simulink model "ES101A_DiagcMgr"  (R2013b)
settings: Solver=ode45  StartTime=0.0  StopTime=0.44  RelTol=1e-3
values from neighbouring files (symbols this model uses):
  BrdgVltg = DataDict.IpSignal    [ES101A_DiagcMgr_DataDict.m]
  DEM_CLEAR_PENDING = DataDict.Constant    [ES101A_DiagcMgr_DataDict.m]
  DEM_DTC_GROUP_ALL_DTCS = DataDict.Constant    [ES101A_DiagcMgr_DataDict.m]
  DFTAGICNTR_CNT_U08 = DataDict.Constant    [ES101A_DiagcMgr_DataDict.m]
  DIAGCMGR_NTCINFOSTSTESTFAILD_CNT_U08 = DataDict.Constant    [ES101A_DiagcMgrProxyX_DataDict.m]    (also in ES101A_DiagcMgr_DataDict.m)
  DIAGCMGR_NTCINFOSTSTESTFAILDTHISIGNCYC_CNT_U08 = DataDict.Constant    [ES101A_DiagcMgr_DataDict.m]
  DIAGCMGR_NTCINFOSTSTESTNOTCMPLTHISIGNCYC_CNT_U08 = DataDict.Constant    [ES101A_DiagcMgrProxyX_DataDict.m]    (also in ES101A_DiagcMgr_DataDict.m)
  DiagcMgrFltResp = DataDict.Calibration    [ES101A_DiagcMgrProxyX_DataDict.m]    (also in ES101A_DiagcMgr_DataDict.m)
  DiagcMgrNtcFltAry = DataDict.NVM    [ES101A_DiagcMgr_DataDict.m]
  DIAGCSTSCTRLDSHTDWNFLTPRSNT_CNT_U16 = DataDict.Constant    [ES101A_DiagcMgr_DataDict.m]
  DIAGCSTSDFTHWAG_CNT_U16 = DataDict.Constant    [ES101A_DiagcMgr_DataDict.m]
  DIAGCSTSDFTHWAGSERLCOMEXPRTVAL_CNT_U16 = DataDict.Constant    [ES101A_DiagcMgr_DataDict.m]
  DIAGCSTSDFTVEHSPD_CNT_U16 = DataDict.Constant    [ES101A_DiagcMgr_DataDict.m]
  DIAGCSTSININVAL_CNT_U16 = DataDict.Constant    [ES101A_DiagcMgrProxyX_DataDict.m]    (also in ES101A_DiagcMgr_DataDict.m)
  DIAGCSTSIVTR1INACTV_CNT_U16 = DataDict.Constant    [ES101A_DiagcMgr_DataDict.m]
  DIAGCSTSIVTR2INACTV_CNT_U16 = DataDict.Constant    [ES101A_DiagcMgr_DataDict.m]
  DIAGCSTSLIMDTPRFMNC_CNT_U16 = DataDict.Constant    [ES101A_DiagcMgr_DataDict.m]
  DIAGCSTSRAMPTOZEROFLTPRSNT_CNT_U16 = DataDict.Constant    [ES101A_DiagcMgr_DataDict.m]
  DIAGCSTSWHLIMBREJCTNDI_CNT_U16 = DataDict.Constant    [ES101A_DiagcMgr_DataDict.m]
  DTCIDXSTSFAIL_CNT_U08 = DataDict.Constant    [ES101A_DiagcMgr_DataDict.m]
  DTCIDXSTSNONTC_CNT_U08 = DataDict.Constant    [ES101A_DiagcMgr_DataDict.m]
  DTCIDXSTSNORES_CNT_U08 = DataDict.Constant    [ES101A_DiagcMgr_DataDict.m]
  DTCIDXSTSPASS_CNT_U08 = DataDict.Constant    [ES101A_DiagcMgr_DataDict.m]
  DTCIDXSTSUPDCFMD_CNT_U08 = DataDict.Constant    [ES101A_DiagcMgr_DataDict.m]
  ELECGLBPRM_IVTRCNT_CNT_U08 = DataDict.ConfigParam    [ES101A_DiagcMgrProxyX_DataDict.m]    (also in ES101A_DiagcMgr_DataDict.m)
  FLTINJ_DIAGCMGR_DIAGCSTSIVTR1INACTV = DataDict.Constant    [ES101A_DiagcMgr_DataDict.m]
  FLTINJ_DIAGCMGR_DIAGCSTSIVTR2INACTV = DataDict.Constant    [ES101A_DiagcMgr_DataDict.m]
  HwTq = DataDict.IpSignal    [ES101A_DiagcMgr_DataDict.m]
  IgnCntr = DataDict.IpSignal    [ES101A_DiagcMgr_DataDict.m]
  MAXDEBCNTRVAL_CNT_S16 = DataDict.Constant    [ES101A_DiagcMgr_DataDict.m]
  MAXRAMPRATE_ULSPERSEC_F32 = DataDict.Constant    [ES101A_DiagcMgrProxyX_DataDict.m]    (also in ES101A_DiagcMgr_DataDict.m)
  MINDEBCNTRVAL_CNT_S16 = DataDict.Constant    [ES101A_DiagcMgr_DataDict.m]
  MINRAMPRATE_ULSPERSEC_F32 = DataDict.Constant    [ES101A_DiagcMgrProxyX_DataDict.m]    (also in ES101A_DiagcMgr_DataDict.m)
  SCAMOTTQCMDTOONE_ULS_F32 = DataDict.Constant    [ES101A_DiagcMgrProxyX_DataDict.m]    (also in ES101A_DiagcMgr_DataDict.m)
  SCAMOTTQCMDTOZERO_ULS_F32 = DataDict.Constant    [ES101A_DiagcMgrProxyX_DataDict.m]    (also in ES101A_DiagcMgr_DataDict.m)
  SysSt = DataDict.IpSignal    [ES101A_DiagcMgr_DataDict.m]
  VehSpd = DataDict.IpSignal    [ES101A_DiagcMgr_DataDict.m]
undefined symbols (not defined in the file or in its folder): ActvMotTqCmdSca, ActvRampRate, AgiCntr, Dem_DTCFormatType, Dem_DTCOriginType, Dem_EventStatusType, DiagcData, DiagcMgrNtcMap, DiagcSts, DtcEnaMask, EcuT, HistNtcFltAry, MicroDiagcData, MotTq, NtcNr, NtcNrWithResd1, NtcStInfo, ProxySetNtcData, Sts, SysSt1, TOTNROFDTC_CNT_U08
libraries: simulink x149, FloatToFixd x5, NxtrNvM x3
(part 8 of 13)

== system ES101A_DiagcMgr/DiagcMgr/SetNtcStsCore/NtcNr is Valid/Diagnostics Not Inhibited/NtcEnabled/NTCSTS_PREFAILD/Update NtcInfoSts, DebCntr and Process RampRate ==
  NtcInfo_ArgIn : Inport
  DebStep_ArgIn : Inport  Port=2
  NtcStInfo_ArgIn : Inport  Port=3
  NtcNr_ArgIn : Inport  Port=4
  DiagcData_ArgIn : Inport  Port=5
  ProxySetNtcData_ArgIn : Inport  Port=6
  NtcInfoDebCntr_ArgIn : Inport  Port=7
  SnapshotDataBus : Inport  Port=8
  Constant : Constant  Value=MAXDEBCNTRVAL_CNT_S16
  CopyRight2 : Subsystem  Description=|  mask(Copyright Information){none=on}
      | Copyright info block.                                               
      |                                                                     
      | Place copyright information at the top of every subsystem in design.
      mask prompts: none "No parameters"
      mask help: Place copyright information at the top of every subsystem in design.
      mask Display:
      | NxtrConf = 'Nexteer Confidential';
      | 
      | sys = bdroot; %handle for the current model ("system")
      | first = get_param(sys,'Created');
      | first = first(end-3:end);  %year is last four digits
      | 
      | last = get_param(sys,'LastModifiedDate');
      | if isempty(last)
      |     last = datestr(now,'yyyy');
      | else
      |     last = last(end-3:end);
      | end
      | 
      | if strcmp(first,last)
      |     fprintf('%s -- Copyright %s Nexteer',NxtrConf,first)
      | else
      |     fprintf('%s -- %s%s- %s Nexteer',NxtrConf,char(169),first,last)
      | end
  Deb Counter < MAXDEBCNTRVAL_CNT_S16 : Subsystem  RequirementInfo="{'linktype_rmi_doors' '0000c474 (/ESG Group/FDD Module Requirements/EA4 Specific/ES101A_DiagcMgr)' '#ES101A_275' 'true' 'REQ:  ES101A_275' '' ; 'linktype_rmi_doors' '0000c474 (/ESG Group/FDD Module Requirements/EA4 Specific/ES101A_DiagcMgr)' '#ES101A_277' 'true' 'REQ:  ES101A_277' '' } %GIDa_78053276_d02e_468e_a567_0a861c97d8c0"  TreatAsAtomicUnit=on
  DebCntr = MAXDEBCNTRVAL_CNT_S16 : Subsystem  TreatAsAtomicUnit=on
  If1 : If  NumInputs=3  IfExpression="(u1 >=  u2) | (u3 >= 32767)"
  Merge1 : Merge
  Sub1 : Sum  Inputs=-+  SaturateOnIntegerOverflow=on
  NtcInfo_ArgOut : Outport
  DiagcData_ArgOut : Outport  Port=2
  NtcInfoDebCntr_ArgOut : Outport  Port=3
  ProxySetNtcData_ArgOut : Outport  Port=4
  wires:
  If1/1 -> DebCntr = MAXDEBCNTRVAL_CNT_S16/Action
  If1/2 -> Deb Counter < MAXDEBCNTRVAL_CNT_S16/Action
  NtcInfo_ArgIn/1 -> Deb Counter < MAXDEBCNTRVAL_CNT_S16/1(NtcInfoDebCntr_ArgIn), DebCntr = MAXDEBCNTRVAL_CNT_S16/5(NtcInfo_ArgIn)
  Constant/1 -> Sub1/2
  Sub1/1 -> If1/2
  Deb Counter < MAXDEBCNTRVAL_CNT_S16/1(NtcInfoDebCntr_ArgOut) -> Merge1/2
  DebCntr = MAXDEBCNTRVAL_CNT_S16/4(NtcInfoDebCntr_ArgOut) -> Merge1/1
  Merge1/1 -> NtcInfoDebCntr_ArgOut/1
  NtcStInfo_ArgIn/1 -> DebCntr = MAXDEBCNTRVAL_CNT_S16/4(NtcStInfo_ArgIn)
  ProxySetNtcData_ArgIn/1 -> DebCntr = MAXDEBCNTRVAL_CNT_S16/3(ProxySetNtcData_ArgIn)
  DiagcData_ArgIn/1 -> DebCntr = MAXDEBCNTRVAL_CNT_S16/2(DiagcData_ArgIn)
  NtcNr_ArgIn/1 -> DebCntr = MAXDEBCNTRVAL_CNT_S16/1(NtcNr_ArgIn)
  DebCntr = MAXDEBCNTRVAL_CNT_S16/1(DiagcData_ArgOut) -> DiagcData_ArgOut/1
  DebCntr = MAXDEBCNTRVAL_CNT_S16/2(ProxySetNtcData_ArgOut) -> ProxySetNtcData_ArgOut/1
  NtcInfoDebCntr_ArgIn/1 -> If1/1
  DebCntr = MAXDEBCNTRVAL_CNT_S16/3(NtcInfo_ArgOut) -> NtcInfo_ArgOut/1
  SnapshotDataBus/1 -> DebCntr = MAXDEBCNTRVAL_CNT_S16/6(SnapshotDataBus)
  DebStep_ArgIn/1 -> Sub1/1, If1/3, Deb Counter < MAXDEBCNTRVAL_CNT_S16/2(DebStep_ArgIn)

== system ES101A_DiagcMgr/DiagcMgr/SetNtcStsCore/NtcNr is Valid/Diagnostics Not Inhibited/NtcEnabled/NTCSTS_PREPASSD/CopyRight2 ==

== system ES101A_DiagcMgr/DiagcMgr/SetNtcStsCore/NtcNr is Valid/Diagnostics Not Inhibited/NtcEnabled/NTCSTS_PREPASSD/Update NtcInfoSts ==
  NtcNr_ArgIn : Inport
  DebStep_ArgIn : Inport  Port=2
  NtcInfo_ArgIn : Inport  Port=3
  NtcInfoDebCntr_ArgIn : Inport  Port=4
  " DIAGCMGR_NTCINFOSTSTESTFAILDTHISIGNCYC_CNT_U08" : simulink/Logic and Bit Operations/Bitwise Operator  logicop=AND  UseBitMask=on  BitMask=DIAGCMGR_NTCINFOSTSTESTFAILDTHISIGNCYC_CNT_U08  BitMaskRealWorld=Stored Integer
  Bus Selector : BusSelector  OutputSignals=Sts
  CopyRight2 : Subsystem  Description=|  mask(Copyright Information){none=on}
      | Copyright info block.                                               
      |                                                                     
      | Place copyright information at the top of every subsystem in design.
      mask prompts: none "No parameters"
      mask help: Place copyright information at the top of every subsystem in design.
      mask Display:
      | NxtrConf = 'Nexteer Confidential';
      | 
      | sys = bdroot; %handle for the current model ("system")
      | first = get_param(sys,'Created');
      | first = first(end-3:end);  %year is last four digits
      | 
      | last = get_param(sys,'LastModifiedDate');
      | if isempty(last)
      |     last = datestr(now,'yyyy');
      | else
      |     last = last(end-3:end);
      | end
      | 
      | if strcmp(first,last)
      |     fprintf('%s -- Copyright %s Nexteer',NxtrConf,first)
      | else
      |     fprintf('%s -- %s%s- %s Nexteer',NxtrConf,char(169),first,last)
      | end
  Data Type Conversion : DataTypeConversion  OutDataTypeStr=boolean
  Data Type Conversion1 : DataTypeConversion  OutDataTypeStr=boolean
  Data Type Conversion2 : DataTypeConversion  OutDataTypeStr=uint16
  Do Nothing : Subsystem
  FLTRESPRCVRLFLT_CNT_U32 : simulink/Logic and Bit Operations/Bitwise Operator  logicop=AND  UseBitMask=on  BitMask=FLTRESPRCVRLFLT_CNT_U32  BitMaskRealWorld=Stored Integer
  Fault Response Table : Constant  Value=DiagcMgrFltResp
  If : If  NumInputs=2  IfExpression=(u1 == 1)|(u2 == 0)
  Selector1 : Selector  IndexMode=Zero-based  InputPortWidth=512  IndexOptions=Index vector (port)  Indices=[1 3]  OutputSizes=1
  Update NTC Info's Status Byte & Update the NTC Fault Array : Subsystem  RequirementInfo="{'linktype_rmi_doors' '0000c474 (/ESG Group/FDD Module Requirements/EA4 Specific/ES101A_DiagcMgr)' '#ES101A_193' 'true' 'REQ:  ES101A_193' '' ; 'linktype_rmi_doors' '0000c474 (/ESG Group/FDD Module Requirements/EA4 Specific/ES101A_DiagcMgr)' '#ES101A_253' 'true' 'REQ:  ES101A_253' '' ; 'linktype_rmi_doors' '0000c474 (/ESG Group/FDD Module Requirements/EA4 Specific/ES101A_DiagcMgr)' '#ES101A_194' 'true' 'REQ:  ES101A_194' '' ; 'linktype_rmi_doors' '0000c474 (/ESG Group/FDD Module Requirements/EA4 Specific/ES101A_DiagcMgr)' '#ES101A_195' 'true' 'REQ:  ES101A_195' '' } %GIDa_8b4eb5db_0f86_4d26_94c4_2021364c827d"
  NtcInfo_ArgOut : Outport
  NtcInfoDebCntr_ArgOut : Outport  Port=2
  wires:
  Data Type Conversion2/1 -> Selector1/2
  Update NTC Info's Status Byte & Update the NTC Fault Array/1("NtcInfo_ArgOut ") -> NtcInfo_ArgOut/1
  Data Type Conversion1/1 -> If/2
  " DIAGCMGR_NTCINFOSTSTESTFAILDTHISIGNCYC_CNT_U08"/1 -> Data Type Conversion1/1
  Bus Selector/1 -> " DIAGCMGR_NTCINFOSTSTESTFAILDTHISIGNCYC_CNT_U08"/1  "<Sts>"
  NtcInfo_ArgIn/1 -> Update NTC Info's Status Byte & Update the NTC Fault Array/1(NtcInfo_ArgIn), Bus Selector/1
  DebStep_ArgIn/1 -> Update NTC Info's Status Byte & Update the NTC Fault Array/2(DebStep_ArgIn)
  If/2 -> Do Nothing/Action
  If/1 -> Update NTC Info's Status Byte & Update the NTC Fault Array/Action
  Data Type Conversion/1 -> If/1
  FLTRESPRCVRLFLT_CNT_U32/1 -> Data Type Conversion/1
  Fault Response Table/1 -> Selector1/1
  Selector1/1 -> FLTRESPRCVRLFLT_CNT_U32/1
  NtcNr_ArgIn/1 -> Data Type Conversion2/1
  NtcInfoDebCntr_ArgIn/1 -> Update NTC Info's Status Byte & Update the NTC Fault Array/3(NtcInfoDebCntr_ArgIn)
  Update NTC Info's Status Byte & Update the NTC Fault Array/2(NtcInfoDebCntr_ArgOut) -> NtcInfoDebCntr_ArgOut/1

== system ES101A_DiagcMgr/DiagcMgr/DiagcMgrIninCore/Update NtcInfoAry From NvM/Update NtcInfoAry/Update NtcInfoAry Aging Counter And Confirmed Bit/If Action/Subsystem/0 < AgingCntr < 64 ==
  note: SW Implementation:
      |
      | 	Design is generalized with the use of "DiagcMgrNtcInfoX" as the NtcInfoAry. When the NTC from the NvM is read
      | 	and it is looked up against the NtcMap to find its ApplIdx and NtcInfoIdx. ApplIdx indicates which NtcInfo the NTC
      | 	belongs to. NtcInfoIdx is used to find the NtcInfo data corresponding to that NTC in the NtcInfoIdx.
      |
      | 	This design does not show which NtcInfoAry does an NTC belong to, instead shows a generalized NtcInfoX.
      | 	The software implementaion shall use the ApplIdx to index into the correct NtcInfoAry and then used the NtcInfoIdx
      | 	to index into the correct data for any NTC.
  NtcNr : Inport
  AgiCntr : Inport  Port=2
  "Sts " : Inport  Port=3
  NtcInfoAry_ArgIn : Inport  Port=4
  Action Port : ActionPort
  Assignment : Assignment  IndexMode=Zero-based  IndexOptions=Index vector (port)  Indices=1  OutputSizes=1
  Bus Assignment1 : BusAssignment  AssignedSignals=Sts,AgiCntr
  Bus Selector2 : BusSelector  OutputSignals=ApplIdx,NtcInfoIdx
  CopyRight2 : Subsystem  Description=|  mask(Copyright Information){none=on}
      | Copyright info block.                                               
      |                                                                     
      | Place copyright information at the top of every subsystem in design.
      mask prompts: none "No parameters"
      mask help: Place copyright information at the top of every subsystem in design.
      mask Display:
      | NxtrConf = 'Nexteer Confidential';
      | 
      | sys = bdroot; %handle for the current model ("system")
      | first = get_param(sys,'Created');
      | first = first(end-3:end);  %year is last four digits
      | 
      | last = get_param(sys,'LastModifiedDate');
      | if isempty(last)
      |     last = datestr(now,'yyyy');
      | else
      |     last = last(end-3:end);
      | end
      | 
      | if strcmp(first,last)
      |     fprintf('%s -- Copyright %s Nexteer',NxtrConf,first)
      | else
      |     fprintf('%s -- %s%s- %s Nexteer',NxtrConf,char(169),first,last)
      | end
  Data Store Read3 : DataStoreRead  DataStoreName=DiagcMgrNtcMap  DataStoreElements=DiagcMgrNtcMap(:)
  Selector : Selector  IndexMode=Zero-based  InputPortWidth=22  IndexOptions=Index vector (port)  Indices=[1 3]  OutputSizes=1
  Selector2 : Selector  IndexMode=Zero-based  InputPortWidth=512  IndexOptions=Index vector (port)  Indices=[1 3]  OutputSizes=1
  Terminator : Terminator
  NtcInfoAry_ArgOut : Outport
  wires:
  AgiCntr/1 -> Bus Assignment1/3
  "Sts "/1 -> Bus Assignment1/2
  Selector2/1 -> Bus Selector2/1
  Data Store Read3/1 -> Selector2/1
  NtcNr/1 -> Selector2/2
  Bus Selector2/2 -> Selector/2, Assignment/3  "<NtcInfoIdx>"
  Selector/1 -> Bus Assignment1/1
  Assignment/1 -> NtcInfoAry_ArgOut/1
  NtcInfoAry_ArgIn/1 -> Assignment/1, Selector/1
  Bus Assignment1/1 -> Assignment/2
  Bus Selector2/1 -> Terminator/1  "<ApplIdx>"

== system ES101A_DiagcMgr/DiagcMgr/DiagcMgrIninCore/Update NtcInfoAry From NvM/Update NtcInfoAry/Update NtcInfoAry Aging Counter And Confirmed Bit/If Action/Subsystem/AgingCntr >= 64 Do Nothing ==
  Action Port : ActionPort
  CopyRight1 : Subsystem  Description=|  mask(Copyright Information){none=on}
      | Copyright info block.                                               
      |                                                                     
      | Place copyright information at the top of every subsystem in design.
      mask prompts: none "No parameters"
      mask help: Place copyright information at the top of every subsystem in design.
      mask Display:
      | NxtrConf = 'Nexteer Confidential';
      | 
      | sys = bdroot; %handle for the current model ("system")
      | first = get_param(sys,'Created');
      | first = first(end-3:end);  %year is last four digits
      | 
      | last = get_param(sys,'LastModifiedDate');
      | if isempty(last)
      |     last = datestr(now,'yyyy');
      | else
      |     last = last(end-3:end);
      | end
      | 
      | if strcmp(first,last)
      |     fprintf('%s -- Copyright %s Nexteer',NxtrConf,first)
      | else
      |     fprintf('%s -- %s%s- %s Nexteer',NxtrConf,char(169),first,last)
      | end

== system ES101A_DiagcMgr/DiagcMgr/DiagcMgrPer2/Clear All DTCs/Call DEM & Update DtcIdxPrevSts/Update DtcIdxPrevSts and PrevClrDtcFlg/Clear All DTCs/For All DTC Indices/CopyRight2 ==

== system ES101A_DiagcMgr/DiagcMgr/DiagcMgrPer2/Normal Periodic Processing/For All DTCs/For Each DTC/Check If DTC Status has Changed/DTC Status Changed OR DTC Update NOT Confirmed/CopyRight2 ==

== system ES101A_DiagcMgr/DiagcMgr/DiagcMgrPer2/Normal Periodic Processing/For All DTCs/For Each DTC/Check If DTC Status has Changed/DTC Status Changed OR DTC Update NOT Confirmed/Update DTC Index Previous Status with DTC Index Current Status ==
  DtcIdx : Inport
  Assignment : Assignment  IndexMode=Zero-based  IndexOptions=Starting index (port)  Indices=1  OutputSizes=1
  CopyRight2 : Subsystem  Description=|  mask(Copyright Information){none=on}
      | Copyright info block.                                               
      |                                                                     
      | Place copyright information at the top of every subsystem in design.
      mask prompts: none "No parameters"
      mask help: Place copyright information at the top of every subsystem in design.
      mask Display:
      | NxtrConf = 'Nexteer Confidential';
      | 
      | sys = bdroot; %handle for the current model ("system")
      | first = get_param(sys,'Created');
      | first = first(end-3:end);  %year is last four digits
      | 
      | last = get_param(sys,'LastModifiedDate');
      | if isempty(last)
      |     last = datestr(now,'yyyy');
      | else
      |     last = last(end-3:end);
      | end
      | 
      | if strcmp(first,last)
      |     fprintf('%s -- Copyright %s Nexteer',NxtrConf,first)
      | else
      |     fprintf('%s -- %s%s- %s Nexteer',NxtrConf,char(169),first,last)
      | end
  Data Store Read : DataStoreRead  DataStoreName=DtcIdxCurrSts
  Data Store Read1 : DataStoreRead  DataStoreName=DtcIdxPrevSts
  Data Store Write : DataStoreWrite  DataStoreName=DtcIdxPrevSts
  wires:
  Assignment/1 -> Data Store Write/1
  DtcIdx/1 -> Assignment/3
  Data Store Read/1 -> Assignment/2
  Data Store Read1/1 -> Assignment/1

== system ES101A_DiagcMgr/DiagcMgr/DiagcMgrPer2/Normal Periodic Processing/For All DTCs/For Each DTC/Check If DTC Status has Changed/DTC Status Changed OR DTC Update NOT Confirmed/Update DTC Status ==
  DtcIdxCurrSts : Inport
  DtcIdx : Inport  Port=2
  CopyRight2 : Subsystem  Description=|  mask(Copyright Information){none=on}
      | Copyright info block.                                               
      |                                                                     
      | Place copyright information at the top of every subsystem in design.
      mask prompts: none "No parameters"
      mask help: Place copyright information at the top of every subsystem in design.
      mask Display:
      | NxtrConf = 'Nexteer Confidential';
      | 
      | sys = bdroot; %handle for the current model ("system")
      | first = get_param(sys,'Created');
      | first = first(end-3:end);  %year is last four digits
      | 
      | last = get_param(sys,'LastModifiedDate');
      | if isempty(last)
      |     last = datestr(now,'yyyy');
      | else
      |     last = last(end-3:end);
      | end
      | 
      | if strcmp(first,last)
      |     fprintf('%s -- Copyright %s Nexteer',NxtrConf,first)
      | else
      |     fprintf('%s -- %s%s- %s Nexteer',NxtrConf,char(169),first,last)
      | end
  Dtc Status is Failed : Subsystem  TreatAsAtomicUnit=on
  Dtc Status is No Result or No Ntc : Subsystem  TreatAsAtomicUnit=on
  Dtc Status is Passed : Subsystem  TreatAsAtomicUnit=on
  If : If  IfExpression=(u1 == 1)  ElseIfExpressions=(u1 == 2)
  wires:
  DtcIdxCurrSts/1 -> If/1
  If/1 -> Dtc Status is Passed/Action
  DtcIdx/1 -> Dtc Status is Failed/1(DtcIdx), Dtc Status is Passed/1(DtcIdx), Dtc Status is No Result or No Ntc/1(DtcIdx)
  If/3 -> Dtc Status is No Result or No Ntc/Action
  If/2 -> Dtc Status is Failed/Action

== system ES101A_DiagcMgr/DiagcMgr/DiagcMgrPer2/Normal Periodic Processing/For All NTCs/For Each NTC/Update DTC Status/NTC Enabled/CopyRight2 ==

== system ES101A_DiagcMgr/DiagcMgr/DiagcMgrPer2/Normal Periodic Processing/For All NTCs/For Each NTC/Update DTC Status/NTC Enabled/DTC Fail ==
  DtcIdx : Inport
  Action Port : ActionPort
  Assignment : Assignment  IndexMode=Zero-based  IndexOptions=Starting index (port)  Indices=1  OutputSizes=1
  CopyRight2 : Subsystem  Description=|  mask(Copyright Information){none=on}
      | Copyright info block.                                               
      |                                                                     
      | Place copyright information at the top of every subsystem in design.
      mask prompts: none "No parameters"
      mask help: Place copyright information at the top of every subsystem in design.
      mask Display:
      | NxtrConf = 'Nexteer Confidential';
      | 
      | sys = bdroot; %handle for the current model ("system")
      | first = get_param(sys,'Created');
      | first = first(end-3:end);  %year is last four digits
      | 
      | last = get_param(sys,'LastModifiedDate');
      | if isempty(last)
      |     last = datestr(now,'yyyy');
      | else
      |     last = last(end-3:end);
      | end
      | 
      | if strcmp(first,last)
      |     fprintf('%s -- Copyright %s Nexteer',NxtrConf,first)
      | else
      |     fprintf('%s -- %s%s- %s Nexteer',NxtrConf,char(169),first,last)
      | end
  DTC Fail : Constant  Value=DTCIDXSTSFAIL_CNT_U08
  Data Store Read : DataStoreRead  DataStoreName=DtcIdxCurrSts
  Data Store Write : DataStoreWrite  DataStoreName=DtcIdxCurrSts
  wires:
  Data Store Read/1 -> Assignment/1
  DTC Fail/1 -> Assignment/2
  Assignment/1 -> Data Store Write/1
  DtcIdx/1 -> Assignment/3

== system ES101A_DiagcMgr/DiagcMgr/DiagcMgrPer2/Normal Periodic Processing/For All NTCs/For Each NTC/Update DTC Status/NTC Enabled/DTC NoRes ==
  DtcIdx : Inport
  Action Port : ActionPort
  Assignment : Assignment  IndexMode=Zero-based  IndexOptions=Starting index (port)  Indices=1  OutputSizes=1
  CopyRight2 : Subsystem  Description=|  mask(Copyright Information){none=on}
      | Copyright info block.                                               
      |                                                                     
      | Place copyright information at the top of every subsystem in design.
      mask prompts: none "No parameters"
      mask help: Place copyright information at the top of every subsystem in design.
      mask Display:
      | NxtrConf = 'Nexteer Confidential';
      | 
      | sys = bdroot; %handle for the current model ("system")
      | first = get_param(sys,'Created');
      | first = first(end-3:end);  %year is last four digits
      | 
      | last = get_param(sys,'LastModifiedDate');
      | if isempty(last)
      |     last = datestr(now,'yyyy');
      | else
      |     last = last(end-3:end);
      | end
      | 
      | if strcmp(first,last)
      |     fprintf('%s -- Copyright %s Nexteer',NxtrConf,first)
      | else
      |     fprintf('%s -- %s%s- %s Nexteer',NxtrConf,char(169),first,last)
      | end
  DTC NoRes : Constant  Value=DTCIDXSTSNORES_CNT_U08
  Data Store Read : DataStoreRead  DataStoreName=DtcIdxCurrSts
  Data Store Write : DataStoreWrite  DataStoreName=DtcIdxCurrSts
  wires:
  Data Store Read/1 -> Assignment/1
  DTC NoRes/1 -> Assignment/2
  Assignment/1 -> Data Store Write/1
  DtcIdx/1 -> Assignment/3

== system ES101A_DiagcMgr/DiagcMgr/DiagcMgrPer2/Normal Periodic Processing/For All NTCs/For Each NTC/Update DTC Status/NTC Enabled/DTC Pass ==
  DtcIdx : Inport
  Action Port : ActionPort
  Assignment : Assignment  IndexMode=Zero-based  IndexOptions=Starting index (port)  Indices=1  OutputSizes=1
  CopyRight2 : Subsystem  Description=|  mask(Copyright Information){none=on}
      | Copyright info block.                                               
      |                                                                     
      | Place copyright information at the top of every subsystem in design.
      mask prompts: none "No parameters"
      mask help: Place copyright information at the top of every subsystem in design.
      mask Display:
      | NxtrConf = 'Nexteer Confidential';
      | 
      | sys = bdroot; %handle for the current model ("system")
      | first = get_param(sys,'Created');
      | first = first(end-3:end);  %year is last four digits
      | 
      | last = get_param(sys,'LastModifiedDate');
      | if isempty(last)
      |     last = datestr(now,'yyyy');
      | else
      |     last = last(end-3:end);
      | end
      | 
      | if strcmp(first,last)
      |     fprintf('%s -- Copyright %s Nexteer',NxtrConf,first)
      | else
      |     fprintf('%s -- %s%s- %s Nexteer',NxtrConf,char(169),first,last)
      | end
  DTC Pass : Constant  Value=DTCIDXSTSPASS_CNT_U08
  Data Store Read : DataStoreRead  DataStoreName=DtcIdxCurrSts
  Data Store Write : DataStoreWrite  DataStoreName=DtcIdxCurrSts
  wires:
  Data Store Read/1 -> Assignment/1
  DTC Pass/1 -> Assignment/2
  Assignment/1 -> Data Store Write/1
  DtcIdx/1 -> Assignment/3

== system ES101A_DiagcMgr/DiagcMgr/DiagcMgrPer2/Normal Periodic Processing/For All NTCs/For Each NTC/Update DTC Status/NTC Enabled/Do Nothing ==
  Action Port : ActionPort
  CopyRight2 : Subsystem  Description=|  mask(Copyright Information){none=on}
      | Copyright info block.                                               
      |                                                                     
      | Place copyright information at the top of every subsystem in design.
      mask prompts: none "No parameters"
      mask help: Place copyright information at the top of every subsystem in design.
      mask Display:
      | NxtrConf = 'Nexteer Confidential';
      | 
      | sys = bdroot; %handle for the current model ("system")
      | first = get_param(sys,'Created');
      | first = first(end-3:end);  %year is last four digits
      | 
      | last = get_param(sys,'LastModifiedDate');
      | if isempty(last)
      |     last = datestr(now,'yyyy');
      | else
      |     last = last(end-3:end);
      | end
      | 
      | if strcmp(first,last)
      |     fprintf('%s -- Copyright %s Nexteer',NxtrConf,first)
      | else
      |     fprintf('%s -- %s%s- %s Nexteer',NxtrConf,char(169),first,last)
      | end

== system ES101A_DiagcMgr/DiagcMgr/DiagcMgrPer2/Normal Periodic Processing/For All NTCs/For Each NTC/Update DTC Status/NTC Enabled/SIGQLFR_FAILD ==
  Action Port : ActionPort
  Passd : Constant  Value=2  OutDataTypeStr=uint8
  NtcQlfr : Outport  InitialOutput=2
  wires:
  Passd/1 -> NtcQlfr/1

== system ES101A_DiagcMgr/DiagcMgr/DiagcMgrPer2/Normal Periodic Processing/For All NTCs/For Each NTC/Update DTC Status/NTC Enabled/SIGQLFR_NORES ==
  Action Port : ActionPort
  NoRes : Constant  Value=0  OutDataTypeStr=uint8
  NtcQlfr : Outport  InitialOutput=0
  wires:
  NoRes/1 -> NtcQlfr/1

== system ES101A_DiagcMgr/DiagcMgr/DiagcMgrPer2/Normal Periodic Processing/For All NTCs/For Each NTC/Update DTC Status/NTC Enabled/SIGQLFR_PASSD ==
  Action Port : ActionPort
  Passd : Constant  OutDataTypeStr=uint8
  NtcQlfr : Outport  InitialOutput=1
  wires:
  Passd/1 -> NtcQlfr/1

== system ES101A_DiagcMgr/DiagcMgr/DiagcMgrPer2/Normal Periodic Processing/For All NTCs/For Each NTC/Update DTC Status/NTC Not Enabled/CopyRight2 ==

== system ES101A_DiagcMgr/DiagcMgr/DiagcMgrPwrDwn/Update NtcFltAry and HistFltAry/For Number of NTCs/Check Aging Counter/Update History Fault Array/If Action Subsystem/CopyRight2 ==

== system ES101A_DiagcMgr/DiagcMgr/ReadNtcFltAry/Update DiagcMgrReadFltInfoAry and HistReadFltAry/For Number of NTCs/Check Aging Counter/Update History Fault Array/If Action Subsystem/CopyRight2 ==

== system ES101A_DiagcMgr/DiagcMgr/SetNtcStsCore/NtcNr is Valid/Diagnostics Not Inhibited/NtcEnabled/NTCSTS_FAILD/Update ISO Bits, Parameter Byte and AgiCntr /CopyRight2 ==

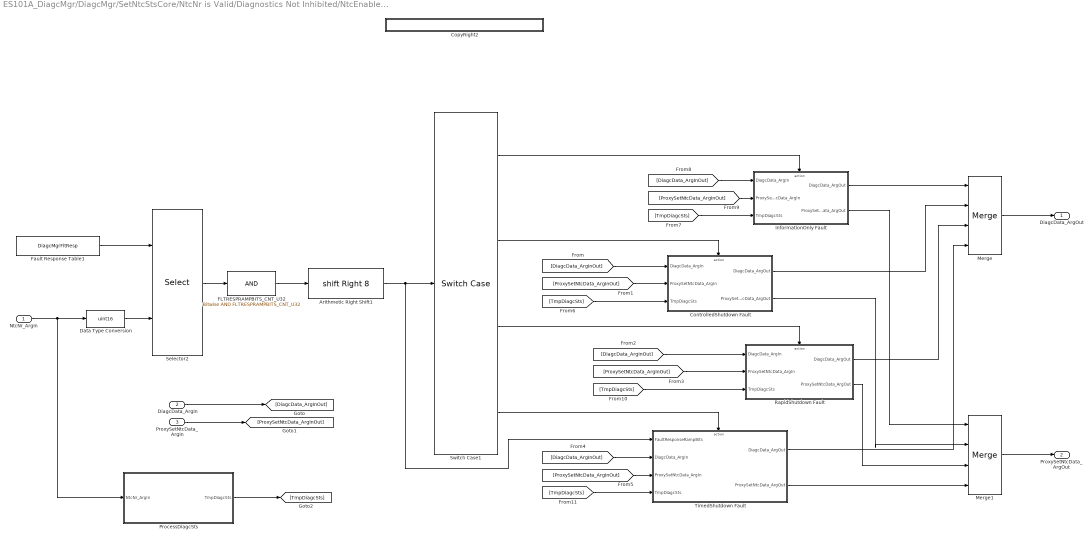
== system ES101A_DiagcMgr/DiagcMgr/SetNtcStsCore/NtcNr is Valid/Diagnostics Not Inhibited/NtcEnabled/NTCSTS_FAILD/Update ISO Bits, Parameter Byte and AgiCntr /ProcessRampResponse and DiagcSts ==
  NtcNr_ArgIn : Inport
  DiagcData_ArgIn : Inport  Port=2
  ProxySetNtcData_ArgIn : Inport  Port=3
  Arithmetic Right Shift1 : ArithShift  BitShiftNumber=8  BitShiftDirection=Right
  ControlledShutdown Fault : Subsystem  RequirementInfo={} %GIDa_c00f0a8c_27b1_40e6_a5b4_93482349b3ad  TreatAsAtomicUnit=on
  CopyRight2 : Subsystem  Description=|  mask(Copyright Information){none=on}
      | Copyright info block.                                               
      |                                                                     
      | Place copyright information at the top of every subsystem in design.
      mask prompts: none "No parameters"
      mask help: Place copyright information at the top of every subsystem in design.
      mask Display:
      | NxtrConf = 'Nexteer Confidential';
      | 
      | sys = bdroot; %handle for the current model ("system")
      | first = get_param(sys,'Created');
      | first = first(end-3:end);  %year is last four digits
      | 
      | last = get_param(sys,'LastModifiedDate');
      | if isempty(last)
      |     last = datestr(now,'yyyy');
      | else
      |     last = last(end-3:end);
      | end
      | 
      | if strcmp(first,last)
      |     fprintf('%s -- Copyright %s Nexteer',NxtrConf,first)
      | else
      |     fprintf('%s -- %s%s- %s Nexteer',NxtrConf,char(169),first,last)
      | end
  Data Type Conversion : DataTypeConversion  OutDataTypeStr=uint16
  FLTRESPRAMPBITS_CNT_U32 : simulink/Logic and Bit Operations/Bitwise Operator  logicop=AND  UseBitMask=on  BitMask=FLTRESPRAMPBITS_CNT_U32  BitMaskRealWorld=Stored Integer
  Fault Response Table1 : Constant  Value=DiagcMgrFltResp
  InformationOnly Fault : Subsystem  RequirementInfo={} %GIDa_dc11e250_3710_463d_b344_07bef256ccac  TreatAsAtomicUnit=on
  Merge : Merge  Inputs=4
  Merge1 : Merge  Inputs=4
  ProcessDiagcSts : Subsystem  RequirementInfo={} %GIDa_1c7e92a4_0b66_42f4_885b_b94fe8d0ca2b
  RapidShutdown Fault : Subsystem  RequirementInfo={} %GIDa_6ebbbb82_fe88_4880_a086_48eed3b76f34  TreatAsAtomicUnit=on
  Selector2 : Selector  IndexMode=Zero-based  InputPortWidth=512  IndexOptions=Index vector (port)  Indices=[1 3]  OutputSizes=1
  Switch Case1 : SwitchCase  CaseConditions={15,14,13}
  TimedShutdown Fault : Subsystem  RequirementInfo={} %GIDa_07f5a547_51e1_4301_a1af_aca0ee87cb19  TreatAsAtomicUnit=on
  DiagcData_ArgOut : Outport
  ProxySetNtcData_ArgOut : Outport  Port=2
  wires:
  NtcNr_ArgIn/1 -> ProcessDiagcSts/1(NtcNr_ArgIn), Data Type Conversion/1
  Arithmetic Right Shift1/1 -> TimedShutdown Fault/1(FaultResponseRampBits), Switch Case1/1
  FLTRESPRAMPBITS_CNT_U32/1 -> Arithmetic Right Shift1/1
  Selector2/1 -> FLTRESPRAMPBITS_CNT_U32/1
  Fault Response Table1/1 -> Selector2/1
  Switch Case1/1 -> InformationOnly Fault/Action
  Switch Case1/2 -> ControlledShutdown Fault/Action
  Switch Case1/3 -> RapidShutdown Fault/Action
  Switch Case1/4 -> TimedShutdown Fault/Action
  Data Type Conversion/1 -> Selector2/2
  DiagcData_ArgIn/1 -> [DiagcData_ArgInOut]
  ProxySetNtcData_ArgIn/1 -> [ProxySetNtcData_ArgInOut]
  [ProxySetNtcData_ArgInOut] -> ControlledShutdown Fault/2(ProxySetNtcData_ArgIn)
  [DiagcData_ArgInOut] -> ControlledShutdown Fault/1(DiagcData_ArgIn)
  [DiagcData_ArgInOut] -> RapidShutdown Fault/1(DiagcData_ArgIn)
  [ProxySetNtcData_ArgInOut] -> RapidShutdown Fault/2(ProxySetNtcData_ArgIn)
  [DiagcData_ArgInOut] -> TimedShutdown Fault/2(DiagcData_ArgIn)
  [ProxySetNtcData_ArgInOut] -> TimedShutdown Fault/3(ProxySetNtcData_ArgIn)
  Merge/1 -> DiagcData_ArgOut/1
  Merge1/1 -> ProxySetNtcData_ArgOut/1
  ProcessDiagcSts/1(TmpDiagcSts) -> [TmpDiagcSts]
  [TmpDiagcSts] -> ControlledShutdown Fault/3(TmpDiagcSts)
  [ProxySetNtcData_ArgInOut] -> InformationOnly Fault/2(ProxySetNtcData_ArgIn)
  [DiagcData_ArgInOut] -> InformationOnly Fault/1(DiagcData_ArgIn)
  [TmpDiagcSts] -> InformationOnly Fault/3(TmpDiagcSts)
  [TmpDiagcSts] -> RapidShutdown Fault/3(TmpDiagcSts)
  [TmpDiagcSts] -> TimedShutdown Fault/4(TmpDiagcSts)
  InformationOnly Fault/1(DiagcData_ArgOut) -> Merge/1
  ControlledShutdown Fault/1(DiagcData_ArgOut) -> Merge/2
  RapidShutdown Fault/1("DiagcData_ArgOut ") -> Merge/3
  TimedShutdown Fault/1(DiagcData_ArgOut) -> Merge/4
  InformationOnly Fault/2(ProxySetNtcData_ArgOut) -> Merge1/1
  ControlledShutdown Fault/2(ProxySetNtcData_ArgOut) -> Merge1/2
  RapidShutdown Fault/2("ProxySetNtcData_ArgOut ") -> Merge1/3
  TimedShutdown Fault/2(ProxySetNtcData_ArgOut) -> Merge1/4

== system ES101A_DiagcMgr/DiagcMgr/SetNtcStsCore/NtcNr is Valid/Diagnostics Not Inhibited/NtcEnabled/NTCSTS_FAILD/Update ISO Bits, Parameter Byte and AgiCntr /UpdSnpshtData ==
  NtcNr : Inport
  NtcStInfo : Inport  Port=2
  SnapshotDataBus : Inport  Port=3
  CopyRight1 : Subsystem  Description=|  mask(Copyright Information){none=on}
      | Copyright info block.                                               
      |                                                                     
      | Place copyright information at the top of every subsystem in design.
      mask prompts: none "No parameters"
      mask help: Place copyright information at the top of every subsystem in design.
      mask Display:
      | NxtrConf = 'Nexteer Confidential';
      | 
      | sys = bdroot; %handle for the current model ("system")
      | first = get_param(sys,'Created');
      | first = first(end-3:end);  %year is last four digits
      | 
      | last = get_param(sys,'LastModifiedDate');
      | if isempty(last)
      |     last = datestr(now,'yyyy');
      | else
      |     last = last(end-3:end);
      | end
      | 
      | if strcmp(first,last)
      |     fprintf('%s -- Copyright %s Nexteer',NxtrConf,first)
      | else
      |     fprintf('%s -- %s%s- %s Nexteer',NxtrConf,char(169),first,last)
      | end
  Data Type Conversion : DataTypeConversion  OutDataTypeStr=uint16
  FLTRESPSNPSHTDATAENAD_CNT_U32 : simulink/Logic and Bit Operations/Bitwise Operator  logicop=AND  UseBitMask=on  BitMask=FLTRESPSNPSHTDATAENAD_CNT_U32  BitMaskRealWorld=Stored Integer
  Fault Response Table1 : Constant  Value=DiagcMgrFltResp
  If : If  IfExpression=u1 ~= 0  ShowElse=off
  Selector2 : Selector  IndexMode=Zero-based  InputPortWidth=512  IndexOptions=Index vector (port)  Indices=[1 3]  OutputSizes=1
  Snapshot Data Enabled : Subsystem
  wires:
  NtcNr/1 -> Snapshot Data Enabled/1(NtcNr), Data Type Conversion/1
  Selector2/1 -> FLTRESPSNPSHTDATAENAD_CNT_U32/1
  Fault Response Table1/1 -> Selector2/1
  Data Type Conversion/1 -> Selector2/2
  NtcStInfo/1 -> Snapshot Data Enabled/2(NtcStInfo)
  SnapshotDataBus/1 -> Snapshot Data Enabled/3(SnapshotDataBus)
  FLTRESPSNPSHTDATAENAD_CNT_U32/1 -> If/1
  If/1 -> Snapshot Data Enabled/Action

== system ES101A_DiagcMgr/DiagcMgr/SetNtcStsCore/NtcNr is Valid/Diagnostics Not Inhibited/NtcEnabled/NTCSTS_FAILD/Update ISO Bits, Parameter Byte and AgiCntr /Update ISO Bits, Parameter Byte and AgiCntr ==
  NtcStInfo_ArgIn : Inport
  NtcInfo_ArgIn : Inport  Port=2
  Bus Assignment1 : BusAssignment  AssignedSignals=Sts,NtcStInfo,AgiCntr
  Bus Selector : BusSelector  OutputSignals=Sts,NtcStInfo
  Clear: DIAGCMGR_NTCINFOSTSTESTNOTCMPLTHISIGNCYC_CNT_U08 : Subsystem
  Constant : Constant  Value=DIAGCMGR_NTCINFOSTSTESTNOTCMPLTHISIGNCYC_CNT_U08
  Constant1 : Constant  Value=0  OutDataTypeStr=uint8
  Constant2 : Constant  Value=MAXDEBCNTRVAL_CNT_S16
  CopyRight2 : Subsystem  Description=|  mask(Copyright Information){none=on}
      | Copyright info block.                                               
      |                                                                     
      | Place copyright information at the top of every subsystem in design.
      mask prompts: none "No parameters"
      mask help: Place copyright information at the top of every subsystem in design.
      mask Display:
      | NxtrConf = 'Nexteer Confidential';
      | 
      | sys = bdroot; %handle for the current model ("system")
      | first = get_param(sys,'Created');
      | first = first(end-3:end);  %year is last four digits
      | 
      | last = get_param(sys,'LastModifiedDate');
      | if isempty(last)
      |     last = datestr(now,'yyyy');
      | else
      |     last = last(end-3:end);
      | end
      | 
      | if strcmp(first,last)
      |     fprintf('%s -- Copyright %s Nexteer',NxtrConf,first)
      | else
      |     fprintf('%s -- %s%s- %s Nexteer',NxtrConf,char(169),first,last)
      | end
  Set Bit: DIAGCMGR_NTCINFOCFMDNTC_CNT_U08 : simulink/Logic and Bit Operations/Bitwise Operator  logicop=OR  UseBitMask=on  BitMask=DIAGCMGR_NTCINFOCFMDNTC_CNT_U08  BitMaskRealWorld=Stored Integer
  Set Bits: DIAGCMGR_NTCINFOSTSTESTFAILDTHISIGNCYC_CNT_U08 : simulink/Logic and Bit Operations/Bitwise Operator  logicop=OR  UseBitMask=on  BitMask=DIAGCMGR_NTCINFOSTSTESTFAILDTHISIGNCYC_CNT_U08  BitMaskRealWorld=Stored Integer
  Set Bits: DIAGCMGR_NTCINFOSTSTESTFAILD_CNT_U08 : simulink/Logic and Bit Operations/Bitwise Operator  logicop=OR  UseBitMask=on  BitMask=DIAGCMGR_NTCINFOSTSTESTFAILD_CNT_U08  BitMaskRealWorld=Stored Integer
  Update NtcStInfo : simulink/Logic and Bit Operations/Bitwise Operator  logicop=OR  UseBitMask=off  NumInputPorts=2  BitMask=bin2dec('11')  BitMaskRealWorld=Stored Integer
  "NtcInfo_ArgOut " : Outport
  NtcInfoDebCntr_ArgOut : Outport  Port=2
  wires:
  Constant1/1 -> Bus Assignment1/4
  Bus Selector/2 -> Update NtcStInfo/1  "<NtcStInfo>"
  Clear: DIAGCMGR_NTCINFOSTSTESTNOTCMPLTHISIGNCYC_CNT_U08/1(Out1) -> Bus Assignment1/2
  Bus Selector/1 -> Set Bits: DIAGCMGR_NTCINFOSTSTESTFAILD_CNT_U08/1  "<Sts>"
  NtcInfo_ArgIn/1 -> Bus Assignment1/1, Bus Selector/1
  Update NtcStInfo/1 -> Bus Assignment1/3
  NtcStInfo_ArgIn/1 -> Update NtcStInfo/2
  Constant/1 -> Clear: DIAGCMGR_NTCINFOSTSTESTNOTCMPLTHISIGNCYC_CNT_U08/2(In1)
  Set Bits: DIAGCMGR_NTCINFOSTSTESTFAILD_CNT_U08/1 -> Set Bits: DIAGCMGR_NTCINFOSTSTESTFAILDTHISIGNCYC_CNT_U08/1
  Set Bits: DIAGCMGR_NTCINFOSTSTESTFAILDTHISIGNCYC_CNT_U08/1 -> Set Bit: DIAGCMGR_NTCINFOCFMDNTC_CNT_U08/1
  Set Bit: DIAGCMGR_NTCINFOCFMDNTC_CNT_U08/1 -> Clear: DIAGCMGR_NTCINFOSTSTESTNOTCMPLTHISIGNCYC_CNT_U08/1(In2)
  Bus Assignment1/1 -> "NtcInfo_ArgOut "/1
  Constant2/1 -> NtcInfoDebCntr_ArgOut/1

== system ES101A_DiagcMgr/DiagcMgr/SetNtcStsCore/NtcNr is Valid/Diagnostics Not Inhibited/NtcEnabled/NTCSTS_PASSD/Update NtcInfoSts /Do Nothing ==
  Action Port : ActionPort  ActionType=else
  CopyRight2 : Subsystem  Description=|  mask(Copyright Information){none=on}
      | Copyright info block.                                               
      |                                                                     
      | Place copyright information at the top of every subsystem in design.
      mask prompts: none "No parameters"
      mask help: Place copyright information at the top of every subsystem in design.
      mask Display:
      | NxtrConf = 'Nexteer Confidential';
      | 
      | sys = bdroot; %handle for the current model ("system")
      | first = get_param(sys,'Created');
      | first = first(end-3:end);  %year is last four digits
      | 
      | last = get_param(sys,'LastModifiedDate');
      | if isempty(last)
      |     last = datestr(now,'yyyy');
      | else
      |     last = last(end-3:end);
      | end
      | 
      | if strcmp(first,last)
      |     fprintf('%s -- Copyright %s Nexteer',NxtrConf,first)
      | else
      |     fprintf('%s -- %s%s- %s Nexteer',NxtrConf,char(169),first,last)
      | end

== system ES101A_DiagcMgr/DiagcMgr/SetNtcStsCore/NtcNr is Valid/Diagnostics Not Inhibited/NtcEnabled/NTCSTS_PASSD/Update NtcInfoSts /Update NTC Info's Status Byte ==
  note: Goes to DebCntr
  NtcInfo_ArgIn : Inport
  Action Port : ActionPort  ActionType=then
  Bus Assignment : BusAssignment  AssignedSignals=Sts
  Bus Selector : BusSelector  OutputSignals=Sts
  Clear: DIAGCMGR_NTCINFOSTSTESTFAILD_CNT_U08 : Subsystem
  Clear: DIAGCMGR_NTCINFOSTSTESTNOTCMPLTHISIGNCYC_CNT_U08 : Subsystem
  Constant : Constant  Value=MINDEBCNTRVAL_CNT_S16
  CopyRight2 : Subsystem  Description=|  mask(Copyright Information){none=on}
      | Copyright info block.                                               
      |                                                                     
      | Place copyright information at the top of every subsystem in design.
      mask prompts: none "No parameters"
      mask help: Place copyright information at the top of every subsystem in design.
      mask Display:
      | NxtrConf = 'Nexteer Confidential';
      | 
      | sys = bdroot; %handle for the current model ("system")
      | first = get_param(sys,'Created');
      | first = first(end-3:end);  %year is last four digits
      | 
      | last = get_param(sys,'LastModifiedDate');
      | if isempty(last)
      |     last = datestr(now,'yyyy');
      | else
      |     last = last(end-3:end);
      | end
      | 
      | if strcmp(first,last)
      |     fprintf('%s -- Copyright %s Nexteer',NxtrConf,first)
      | else
      |     fprintf('%s -- %s%s- %s Nexteer',NxtrConf,char(169),first,last)
      | end
  Test Failed : Constant  Value=DIAGCMGR_NTCINFOSTSTESTFAILD_CNT_U08
  Test Not Complete This Ignition Cycle : Constant  Value=DIAGCMGR_NTCINFOSTSTESTNOTCMPLTHISIGNCYC_CNT_U08
  NtcInfo_ArgOut : Outport
  NtcInfoDebCntr_ArgOut : Outport  Port=2
  wires:
  Test Not Complete This Ignition Cycle/1 -> Clear: DIAGCMGR_NTCINFOSTSTESTNOTCMPLTHISIGNCYC_CNT_U08/2(In1)
  Test Failed/1 -> Clear: DIAGCMGR_NTCINFOSTSTESTFAILD_CNT_U08/2(In1)
  Clear: DIAGCMGR_NTCINFOSTSTESTFAILD_CNT_U08/1(Out1) -> Clear: DIAGCMGR_NTCINFOSTSTESTNOTCMPLTHISIGNCYC_CNT_U08/1(In2)
  Bus Selector/1 -> Clear: DIAGCMGR_NTCINFOSTSTESTFAILD_CNT_U08/1(In2)  "<Sts>"
  Bus Assignment/1 -> NtcInfo_ArgOut/1
  Clear: DIAGCMGR_NTCINFOSTSTESTNOTCMPLTHISIGNCYC_CNT_U08/1(Out1) -> Bus Assignment/2
  NtcInfo_ArgIn/1 -> Bus Assignment/1, Bus Selector/1
  Constant/1 -> NtcInfoDebCntr_ArgOut/1

== system ES101A_DiagcMgr/DiagcMgr/SetNtcStsCore/NtcNr is Valid/Diagnostics Not Inhibited/NtcEnabled/NTCSTS_PREFAILD/Update NtcInfoSts, DebCntr and Process RampRate/CopyRight2 ==

== system ES101A_DiagcMgr/DiagcMgr/SetNtcStsCore/NtcNr is Valid/Diagnostics Not Inhibited/NtcEnabled/NTCSTS_PREFAILD/Update NtcInfoSts, DebCntr and Process RampRate/Deb Counter < MAXDEBCNTRVAL_CNT_S16 ==
  NtcInfoDebCntr_ArgIn : Inport
  DebStep_ArgIn : Inport  Port=2
  Action Port : ActionPort
  Copyright1 : Subsystem  Description=|  mask(Copyright Information){none=on}
      | Copyright info block.                                               
      |                                                                     
      | Place copyright information at the top of every subsystem in design.
      mask prompts: none "No parameters"
      mask help: Place copyright information at the top of every subsystem in design.
      mask Display:
      | NxtrConf = 'Nexteer Confidential';
      | 
      | sys = bdroot; %handle for the current model ("system")
      | first = get_param(sys,'Created');
      | if(isempty(first))
      |     first = datestr(now,'yyyy');
      | else
      |     first = first(end-3:end);  %year is last four digits
      | end
      | 
      | last = get_param(sys,'LastModifiedDate');
      | if isempty(last)
      |     last = datestr(now,'yyyy');
      | else
      |     last = last(end-3:end);
      | end
      | 
      | if strcmp(first,last)
      |     fprintf('%s\nCopyright  %s Nexteer',NxtrConf,first);
      | else
      |     fprintf('%s\n%s%s-%s Nexteer',NxtrConf,char(169),first,last);
      | end
  DebCntr = DebCntr + DebStep : Subsystem
  DebCntr = DebStep : Subsystem  TreatAsAtomicUnit=on
  If : If  IfExpression=u1 < 0
  Merge : Merge
  NtcInfoDebCntr_ArgOut : Outport
  wires:
  NtcInfoDebCntr_ArgIn/1 -> If/1, DebCntr = DebCntr + DebStep/2(NtcInfoDebCntr_ArgIn)
  DebStep_ArgIn/1 -> DebCntr = DebCntr + DebStep/1(DebStep_ArgIn), DebCntr = DebStep/1(DebStep_ArgIn)
  If/1 -> DebCntr = DebStep/Action
  If/2 -> DebCntr = DebCntr + DebStep/Action
  DebCntr = DebStep/1(NtcInfoDebCntr_ArgOut) -> Merge/1
  DebCntr = DebCntr + DebStep/1(NtcInfoDebCntr_ArgOut) -> Merge/2
  Merge/1 -> NtcInfoDebCntr_ArgOut/1

== system ES101A_DiagcMgr/DiagcMgr/SetNtcStsCore/NtcNr is Valid/Diagnostics Not Inhibited/NtcEnabled/NTCSTS_PREFAILD/Update NtcInfoSts, DebCntr and Process RampRate/DebCntr = MAXDEBCNTRVAL_CNT_S16 ==
  NtcNr_ArgIn : Inport
  DiagcData_ArgIn : Inport  Port=2
  ProxySetNtcData_ArgIn : Inport  Port=3
  NtcStInfo_ArgIn : Inport  Port=4
  NtcInfo_ArgIn : Inport  Port=5
  SnapshotDataBus : Inport  Port=6
  Action Port : ActionPort
  Copyright1 : Subsystem  Description=|  mask(Copyright Information){none=on}
      | Copyright info block.                                               
      |                                                                     
      | Place copyright information at the top of every subsystem in design.
      mask prompts: none "No parameters"
      mask help: Place copyright information at the top of every subsystem in design.
      mask Display:
      | NxtrConf = 'Nexteer Confidential';
      | 
      | sys = bdroot; %handle for the current model ("system")
      | first = get_param(sys,'Created');
      | if(isempty(first))
      |     first = datestr(now,'yyyy');
      | else
      |     first = first(end-3:end);  %year is last four digits
      | end
      | 
      | last = get_param(sys,'LastModifiedDate');
      | if isempty(last)
      |     last = datestr(now,'yyyy');
      | else
      |     last = last(end-3:end);
      | end
      | 
      | if strcmp(first,last)
      |     fprintf('%s\nCopyright  %s Nexteer',NxtrConf,first);
      | else
      |     fprintf('%s\n%s%s-%s Nexteer',NxtrConf,char(169),first,last);
      | end
  ProcessRampResponse and DiagcSts : Subsystem  RequirementInfo="{'linktype_rmi_doors' '0000c474 (/ESG Group/FDD Module Requirements/EA4 Specific/ES101A_DiagcMgr)' '#ES101A_73' 'true' 'REQ:  ES101A_73' '' ; 'linktype_rmi_doors' '0000c474 (/ESG Group/FDD Module Requirements/EA4 Specific/ES101A_DiagcMgr)' '#ES101A_290' 'true' 'REQ:  ES101A_290' '' } %GIDa_52772de1_9241_407b_bf6c_3248aa2c1842"
  UpdSnpshtData : Subsystem  RequirementInfo="{'linktype_rmi_doors' '0000c474 (/ESG Group/FDD Module Requirements/EA4 Specific/ES101A_DiagcMgr)' '#ES101A_327' 'true' 'REQ:  ES101A_327' '' ; 'linktype_rmi_doors' '0000c474 (/ESG Group/FDD Module Requirements/EA4 Specific/ES101A_DiagcMgr)' '#ES101A_329' 'true' 'REQ:  ES101A_329' '' ; 'linktype_rmi_doors' '0000c474 (/ESG Group/FDD Module Requirements/EA4 Specific/ES101A_DiagcMgr)' '#ES101A_338' 'true' 'REQ:  ES101A_338' '' } %GIDa_ff276e38_1458_4e36_ab67_a5ffc67bcf13"
  Update NtcSts and DebCntr : Subsystem  RequirementInfo="{'linktype_rmi_doors' '0000c474 (/ESG Group/FDD Module Requirements/EA4 Specific/ES101A_DiagcMgr)' '#ES101A_169' 'true' 'REQ:  ES101A_169' '' ; 'linktype_rmi_doors' '0000c474 (/ESG Group/FDD Module Requirements/EA4 Specific/ES101A_DiagcMgr)' '#ES101A_189' 'true' 'REQ:  ES101A_189' '' ; 'linktype_rmi_doors' '0000c474 (/ESG Group/FDD Module Requirements/EA4 Specific/ES101A_DiagcMgr)' '#ES101A_251' 'true' 'REQ:  ES101A_251' '' ; 'linktype_rmi_doors' '0000c474 (/ESG Group/FDD Module Requirements/EA4 Specific/ES101A_DiagcMgr)' '#ES101A_190' 'true' 'REQ:  ES101A_190' '' ; 'linktype_rmi_doors' '0000c474 (/ESG Group/FDD Module Requirements/EA4 Specific/ES101A_DiagcMgr)' '#ES101A_191' 'true' 'REQ:  ES101A_191' '' } %GIDa_0fa7bac5_ec43_4ad6_9b33_1a7aa2ea96c9"
  DiagcData_ArgOut : Outport
  ProxySetNtcData_ArgOut : Outport  Port=2
  NtcInfo_ArgOut : Outport  Port=3
  NtcInfoDebCntr_ArgOut : Outport  Port=4
  wires:
  ProxySetNtcData_ArgIn/1 -> ProcessRampResponse and DiagcSts/3(ProxySetNtcData_ArgIn)
  NtcNr_ArgIn/1 -> UpdSnpshtData/1(NtcNr), ProcessRampResponse and DiagcSts/1(NtcNr_ArgIn)
  DiagcData_ArgIn/1 -> ProcessRampResponse and DiagcSts/2(DiagcData_ArgIn)
  NtcInfo_ArgIn/1 -> UpdSnpshtData/2(NtcStInfo), Update NtcSts and DebCntr/1(NtcInfo_ArgIn)
  Update NtcSts and DebCntr/1(NtcInfo_ArgOut) -> NtcInfo_ArgOut/1
  NtcStInfo_ArgIn/1 -> Update NtcSts and DebCntr/2(NtcStInfo_ArgIn)
  ProcessRampResponse and DiagcSts/1(DiagcData_ArgOut) -> DiagcData_ArgOut/1
  ProcessRampResponse and DiagcSts/2(ProxySetNtcData_ArgOut) -> ProxySetNtcData_ArgOut/1
  Update NtcSts and DebCntr/2(NtcInfoDebCntr_ArgOut) -> NtcInfoDebCntr_ArgOut/1
  SnapshotDataBus/1 -> UpdSnpshtData/3(SnapshotDataBus)

== system ES101A_DiagcMgr/DiagcMgr/SetNtcStsCore/NtcNr is Valid/Diagnostics Not Inhibited/NtcEnabled/NTCSTS_PREPASSD/Update NtcInfoSts/CopyRight2 ==
